simulink model "InjVlv_CalcET"  (R2020b)
settings: configuration reference "cs_ert" (kept outside this file)
values from neighbouring files (symbols this model uses):
  InjVlv_tiET_MAP = 0.0 0.0 0.0 0.0 0.0 0.0 0.0 0.0 0.0 0.0 0.0 0.0 0.0 0.0 0.0 0.0 414.0 362.4 311.2 267.2 252.0 237.6 230.4 222.8 222.8 222.8 222.8 222.8 222.8 218.4 218.4 208.4 509.6 450.8 392.0 303.6 281.6 267.2 259.6 252.4 244.8 244.8 244.8 237.6 230.4 230.4 230.4 222.8 622.8 553.6 484.4 392.0 318.4 296.4 284.0 274.4 267.2 267.2 259.6 252.4 252.4 244.8 244.8 237.6 733.2 634.4 536.0 443.6 384.8 348.8 311.2 296.4    [InjVlv_CalcET.sldd]
  InjVlv_tiET_MAPX : value not decoded    [InjVlv_CalcET.sldd]
  InjVlv_tiET_MAPY : value not decoded    [InjVlv_CalcET.sldd]
  SigTst_swtMI1ET_C = 0    [InjVlv_CalcET.sldd]
  SigTst_tiMI1ET_C = 0.0    [InjVlv_CalcET.sldd]
undefined symbols (not defined in the file or in its folder): CEngDst_switch_conv, Switch
settings Model: DataDictionary=InjVlv_CalcET.sldd  EnableAccessToBaseWorkspace=off  Creator=zhoutinglin  LastModifiedBy=zhoutinglin
settings ConfigSetRef: SourceName=cs_ert

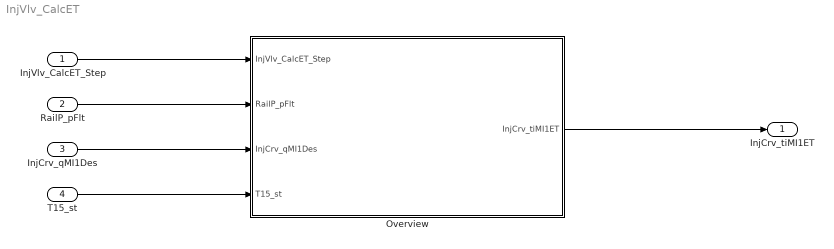
== system InjVlv_CalcET ==
  InjVlv_CalcET_Step : Inport  OutputFunctionCall=on
  RailP_pFlt : Inport  Description=Maximum rail pressure of the last 10 sampling cycle  Port=2  OutMin=0  OutMax=2000  OutDataTypeStr=Press_bar1  Unit=bar  PortDimensions=[1 1]
  InjCrv_qMI1Des : Inport  Description=desired MI1 injection quantity  Port=3  OutMin=-319  OutMax=319  OutDataTypeStr=InjMass  Unit=mg/hub  PortDimensions=[1 1]
  T15_st : Inport  Description=Terminal 15 status after debouncing  Port=4  OutDataTypeStr=Enum:Switch  PortDimensions=[1 1]
  Overview : Subsystem
  InjCrv_tiMI1ET : Outport  Description=Estimated MI1 energizing time  OutMin=-13107  OutMax=13106  OutDataTypeStr=uSec4  Unit=us  PortDimensions=[1 1]
  wires:
  InjVlv_CalcET_Step/1 -> Overview/1(InjVlv_CalcET_Step)
  RailP_pFlt/1 -> Overview/2(RailP_pFlt)
  InjCrv_qMI1Des/1 -> Overview/3(InjCrv_qMI1Des)
  T15_st/1 -> Overview/4(T15_st)
  Overview/1(InjCrv_tiMI1ET) -> InjCrv_tiMI1ET/1

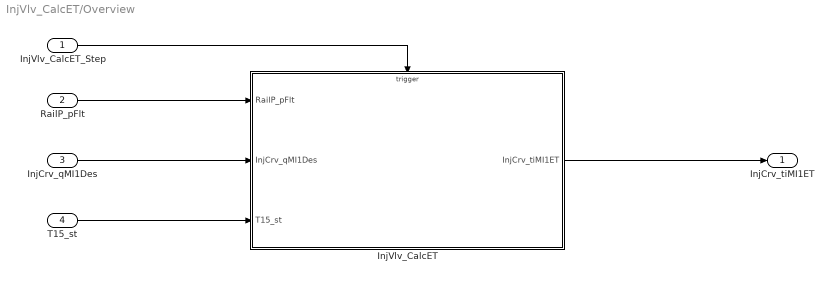
== system InjVlv_CalcET/Overview ==
  InjVlv_CalcET_Step : Inport
  RailP_pFlt : Inport  Port=2
  InjCrv_qMI1Des : Inport  Port=3
  T15_st : Inport  Port=4
  InjVlv_CalcET : Subsystem
  InjCrv_tiMI1ET : Outport  VectorParamsAs1DForOutWhenUnconnected=off
  wires:
  RailP_pFlt/1 -> InjVlv_CalcET/1(RailP_pFlt)
  InjCrv_qMI1Des/1 -> InjVlv_CalcET/2(InjCrv_qMI1Des)
  T15_st/1 -> InjVlv_CalcET/3(T15_st)
  InjVlv_CalcET/1(InjCrv_tiMI1ET) -> InjCrv_tiMI1ET/1
  InjVlv_CalcET_Step/1 -> InjVlv_CalcET/Trigger

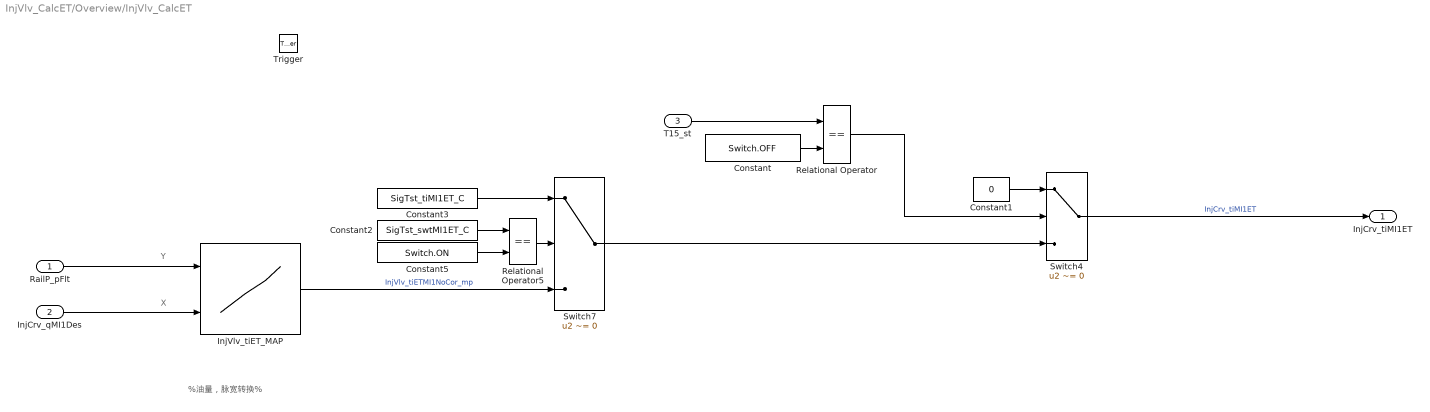
== system InjVlv_CalcET/Overview/InjVlv_CalcET ==
  note: %油量，脉宽转换%
  note: X
  note: Y
  RailP_pFlt : Inport  Tag=bar
  InjCrv_qMI1Des : Inport  Tag=mg/hub  Port=2
  T15_st : Inport  Port=3
  Trigger : TriggerPort  TriggerType=function-call  VariantControl=Variant  PortDimensions=1
  Constant : Constant  Value=Switch.OFF
  Constant1 : Constant  Value=0  OutDataTypeStr=Inherit: Inherit via back propagation
  Constant2 : Constant  Value=SigTst_swtMI1ET_C  SampleTime=-1
  Constant3 : Constant  Value=SigTst_tiMI1ET_C  SampleTime=-1
  Constant5 : Constant  Value=Switch.ON  OutDataTypeStr=Inherit: Inherit via back propagation
  InjVlv_tiET_MAP : Lookup_n-D  BreakpointsForDimension1=InjVlv_tiET_MAPY  BreakpointsForDimension2=InjVlv_tiET_MAPX  IndexSearchMethod=Linear search  BeginIndexSearchUsingPreviousIndexResult=on  Table=InjVlv_tiET_MAP  ExtrapMethod=Clip  UseLastTableValue=on  InternalRulePriority=Speed  OutDataTypeStr=Inherit: Inherit via back propagation  SaturateOnIntegerOverflow=on
      settings: InputPortMap=u0,u1
  Relational Operator : RelationalOperator  Operator===  OutDataTypeStr=boolean  RndMeth=Simplest
  Relational Operator5 : RelationalOperator  Operator===  OutDataTypeStr=boolean  RndMeth=Simplest  InputSameDT=on
  Switch4 : Switch  Criteria=u2 ~= 0  InputSameDT=on
  Switch7 : Switch  Criteria=u2 ~= 0  Threshold=CEngDst_switch_conv.OFF  InputSameDT=on
  InjCrv_tiMI1ET : Outport  Tag=us  VectorParamsAs1DForOutWhenUnconnected=off
  wires:
  Constant/1 -> Relational Operator/2
  Switch7/1 -> Switch4/3
  Constant5/1 -> Relational Operator5/2
  Relational Operator/1 -> Switch4/2
  Relational Operator5/1 -> Switch7/2
  Constant2/1 -> Relational Operator5/1
  Constant1/1 -> Switch4/1
  Switch4/1 -> InjCrv_tiMI1ET/1  "InjCrv_tiMI1ET"
  Constant3/1 -> Switch7/1
  T15_st/1 -> Relational Operator/1
  RailP_pFlt/1 -> InjVlv_tiET_MAP/1
  InjVlv_tiET_MAP/1 -> Switch7/3  "InjVlv_tiETMI1NoCor_mp"
  InjCrv_qMI1Des/1 -> InjVlv_tiET_MAP/2
